simulink model "LQR_sim"  (R2022a)
settings: Solver=VariableStepAuto  StartTime=0.0  StopTime=10  RelTol=1e-3
undefined symbols (not defined in the file): A, B, C, D, K_i_lq, K_s_lq
settings Model: Creator=valen  LastModifiedBy=valen

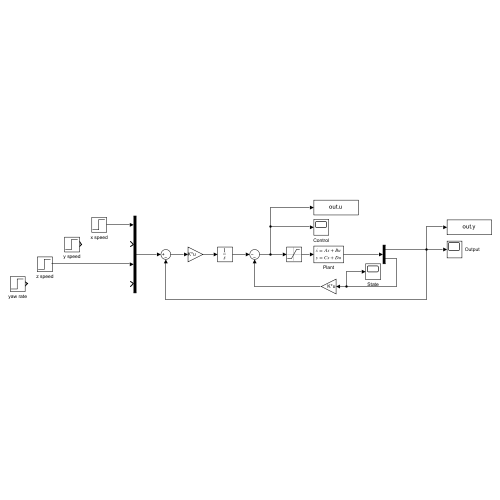
[thumbnail: Simulink's stored preview of the top-level diagram]
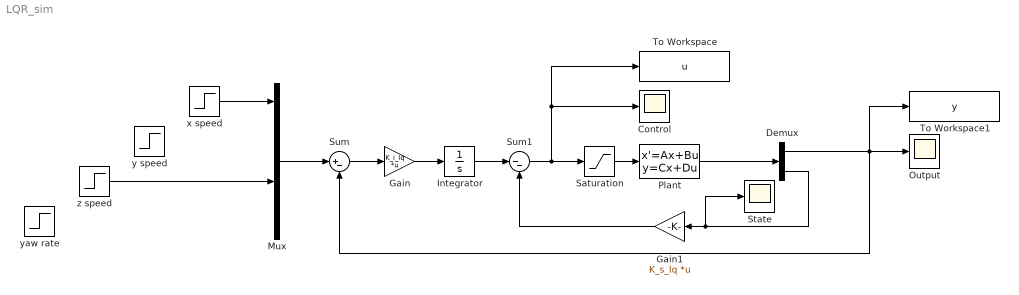
== system LQR_sim ==
  Control : Scope
  Demux : Demux  Outputs=[4, 13]
  Gain : Gain  Gain=K_i_lq  Multiplication=Matrix(K*u)
  Gain1 : Gain  Gain=K_s_lq  Multiplication=Matrix(K*u)
  Integrator : Integrator
  Mux : Mux
  Output : Scope
  Plant : StateSpace  A=A  B=B  C=[C; eye(13)]  D=[D;zeros(13,4)]  InitialCondition=0
  Saturation : Saturate  UpperLimit=1  LowerLimit=-1
  State : Scope
  Sum : Sum  Inputs=|+-
  Sum1 : Sum  Inputs=|--
  To Workspace : ToWorkspace  VariableName=u  SaveFormat=Structure With Time  SampleTime=-1
  To Workspace1 : ToWorkspace  VariableName=y  SaveFormat=Structure With Time  SampleTime=-1
  x speed : Step  Time=0  SampleTime=0
  y speed : Step  Time=0  SampleTime=0
  yaw rate : Step  Time=0  SampleTime=0
  z speed : Step  Time=3  After=0.5  SampleTime=0
  wires:
  Integrator/1 -> Sum1/1
  Gain1/1 -> Sum1/2
  Gain/1 -> Integrator/1
  Sum/1 -> Gain/1
  Demux/2 -> State/1, Gain1/1
  Plant/1 -> Demux/1
  Mux/1 -> Sum/1
  x speed/1 -> Mux/1
  z speed/1 -> Mux/3
  Saturation/1 -> Plant/1
  Sum1/1 -> Saturation/1, To Workspace/1, Control/1
  Demux/1 -> Output/1, To Workspace1/1, Sum/2
